simulink model "controlArduino_Uno_DIO"  (R2023a)
settings: Solver=ode3  StartTime=0.0  StopTime=inf  FixedStep=0.01  RelTol=1e-3  EnableMultiTasking=on
libraries: arduinolib x4, simulink x1
settings Model: ExtModeTrigDuration=2  Creator=The MathWorks, Inc.  LastModifiedBy=ppatel
settings SolverCC: AlgebraicLoopSolver=TrustRegion
settings DataIOCC: LimitDataPoints=on  SaveFormat=Array
settings OptimizationCC: ExpressionDepthLimit=2147483647  LifeSpan=Inf  MaxStackSize=64
settings DebuggingCC: UnconnectedInputMsg=warning  UnconnectedOutputMsg=warning  UnconnectedLineMsg=warning  AllowSymbolicDim=off  StateNameClashWarn=warning  SFUnexpectedBacktrackingDiag=warning  SFNoUnconditionalDefaultTransitionDiag=warning  SFExecutionAtInitializationDiag=none  ArithmeticOperatorsInVariantConditions=warning
settings HardwareCC: ProdBitPerInt=16  ProdBitPerPointer=16  ProdBitPerSizeT=16  ProdBitPerPtrDiffT=16  ProdLargestAtomicFloat=None  ProdWordSize=8  ProdHWDeviceType=Atmel->AVR
settings ModelReferenceCC: EnableRefExpFcnMdlSchedulingChecks=on  PropagateSignalLabelsOutOfModel=off
settings SFSimCC: SimUseLocalCustomCode=off  MATLABDynamicMemAlloc=off
settings RTWCC: Description=Embedded Coder  SystemTargetFile=ert.tlc  HardwareBoard=Arduino Uno  TemplateMakefile=ert_default_tmf  GenerateReport=on  RTWVerbose=off  RTWUseLocalCustomCode=off  Toolchain=Arduino AVR  BuildConfiguration=Faster Runs  LaunchReport=on
settings CodeAppCC: ForceParamTrailComments=on  OperatorAnnotations=on  StateflowObjectComments=on  MATLABSourceComments=on
settings ERTTargetCC: MultiwordLength=2048  ERTCustomFileBanners=off  SupportContinuousTime=on  SupportNonInlinedSFcns=on  RemoveResetFunc=off  SupportVariableSizeSignals=on  ModelStepFunctionPrototypeControlCompliant=off  ExtModeTransport=3  ExtModeStaticAlloc=on  ExtModeAutomaticAllocSize=off  ExtModeStaticAllocSize=250  ExtModeMexFile=ext_xcp  ExtModeIntrfLevel=Level2 - Open
settings ConfigComp: CovMetricSettings=dw  CovSaveCumulativeToWorkspaceVar=on  CovSaveSingleToWorkspaceVar=on  CovExternalEMLEnable=off  CovSFcnEnable=off

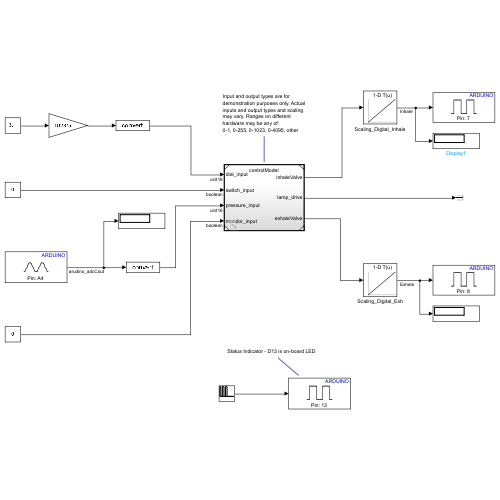
[thumbnail: Simulink's stored preview of the top-level diagram]
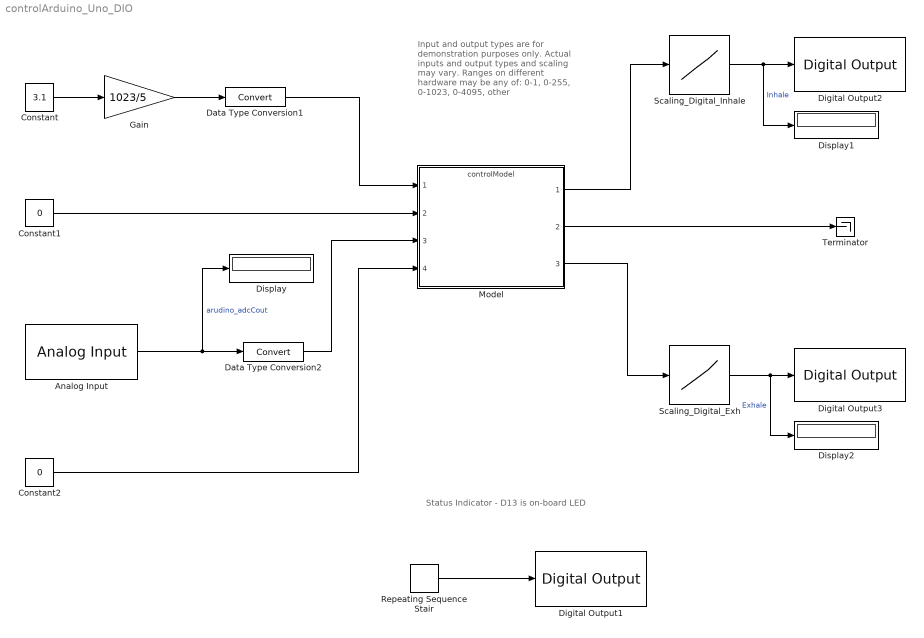
== system controlArduino_Uno_DIO ==
  note: Status Indicator - D13 is on-board LED
  note: Input and output types are for
      | demonstration purposes only. Actual
      | inputs and output types and scaling
      | may vary. Ranges on different
      | hardware may be any of:
      | 0-1, 0-255, 0-1023, 0-4095, other
  Analog Input : arduinolib/Analog Input  pinNumber=4  ReadResultsOnly=off  ConversionTriggerSource=Software  ExternalTriggerType=uint32(0)  OutputDataType=uint16  EnableConversionCompleteNotify=off  EnableOuputStatus=off  SampleTime=-1  blockPlatform=arduino
  Constant : Constant  Value=3.1
  Constant1 : Constant  Value=0  OutDataTypeStr=boolean
  Constant2 : Constant  Value=0  OutDataTypeStr=boolean
  Data Type Conversion1 : DataTypeConversion  RndMeth=Floor
  Data Type Conversion2 : DataTypeConversion  RndMeth=Floor
  Digital Output1 : arduinolib/Digital Output  pinNumber=13  Direction=output  blockPlatform=arduino
  Digital Output2 : arduinolib/Digital Output  pinNumber=7  Direction=output  blockPlatform=arduino
  Digital Output3 : arduinolib/Digital Output  pinNumber=8  Direction=output  blockPlatform=arduino
  Display : Display
  Display1 : Display
  Display2 : Display
  Gain : Gain  Gain=1023/5  OutDataTypeStr=uint16
  Model : ModelReference  ModelNameDialog=controlModel  SimulationMode=Normal  ModelReferenceVersion=8.8
  Repeating Sequence Stair : simulink/Sources/Repeating Sequence Stair  OutValues=[1 0 1 0 1 0 0 0 0 0].'  tsamp=0.2  OutMin=[]  OutMax=[]  OutDataTypeStr=double  OutputDataTypeScalingMode=double  OutDataType=fixdt(0,8)  ConRadixGroup=Best Precision: Vector-wise  OutScaling=2^-12
  Scaling_Digital_Exh : Lookup_n-D  NumberOfTableDimensions=1  BreakpointsForDimension1=[0 255]  BreakpointsForDimension1DataTypeStr=double  Table=[0 1]  TableDataTypeStr=Inherit: Inherit from 'Table data'  ExtrapMethod=Clip  InternalRulePriority=Speed  OutDataTypeStr=Inherit: Inherit via back propagation  RndMeth=Simplest
  Scaling_Digital_Inhale : Lookup_n-D  NumberOfTableDimensions=1  BreakpointsForDimension1=[0 89]  BreakpointsForDimension1DataTypeStr=double  Table=[0 1]  TableDataTypeStr=Inherit: Inherit from 'Table data'  ExtrapMethod=Clip  InternalRulePriority=Speed  OutDataTypeStr=Inherit: Inherit via back propagation  RndMeth=Simplest
  Terminator : Terminator
  wires:
  Model/2 -> Terminator/1
  Gain/1 -> Data Type Conversion1/1
  Constant2/1 -> Model/4
  Constant1/1 -> Model/2
  Repeating Sequence Stair/1 -> Digital Output1/1
  Constant/1 -> Gain/1
  Data Type Conversion2/1 -> Model/3
  Data Type Conversion1/1 -> Model/1
  Model/1 -> Scaling_Digital_Inhale/1
  Model/3 -> Scaling_Digital_Exh/1
  Scaling_Digital_Inhale/1 -> Digital Output2/1, Display1/1  "Inhale"
  Scaling_Digital_Exh/1 -> Display2/1, Digital Output3/1  "Exhale"
  Analog Input/1 -> Display/1, Data Type Conversion2/1  "arudino_adcCout"
